simulink model "mdlspol2pop"  (Simulink 7.8)
settings: Solver=ode45  StartTime=0.0  StopTime=500  RelTol=1e-3
settings Model: Creator=polacmi1  LastModifiedBy=polacekm
settings GRTTargetCC: CombineOutputUpdateFcns=on

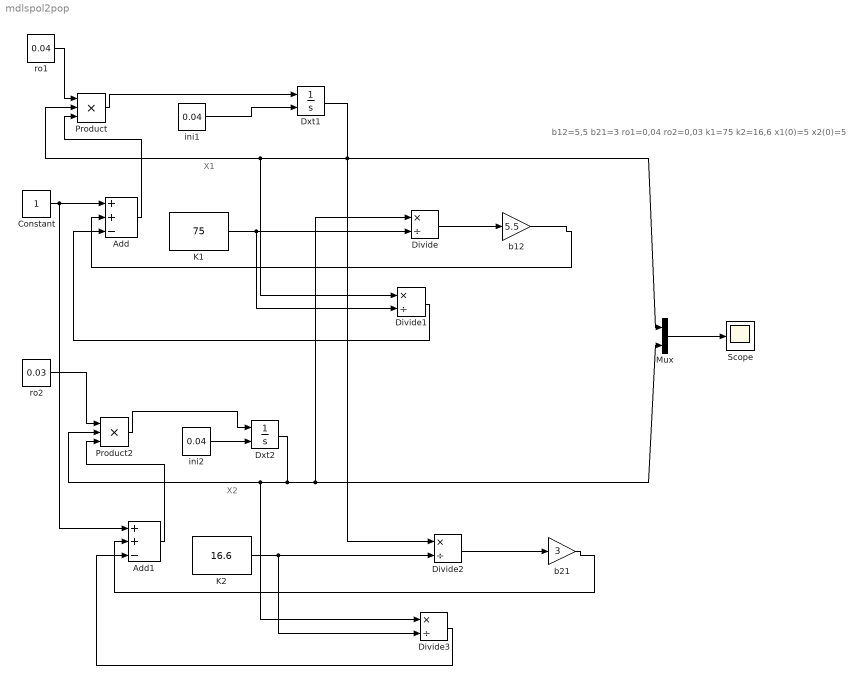
== system mdlspol2pop ==
  note: X1
  note: X2
  note: b12=5,5
      | b21=3
      | ro1=0,04
      | ro2=0,03
      | k1=75
      | k2=16,6
      | x1(0)=5
      | x2(0)=5
  Add : Sum  Inputs=++-
  Add1 : Sum  Inputs=++-
  Constant : Constant
  Divide{,1..3} (4 alike) : Product  Inputs=*/
  Dxt1 : Integrator  InitialConditionSource=external  InitialCondition=10
  Dxt2 : Integrator  InitialConditionSource=external  InitialCondition=10
  K1 : Constant  Value=75
  K2 : Constant  Value=16.6
  Mux : Mux  Inputs=2
  Product : Product  Inputs=3  RndMeth=Zero
  Product2 : Product  Inputs=3  RndMeth=Zero
  Scope : Scope
      settings: SaveName=sc
  b12 : Gain  Gain=5.5
  b21 : Gain  Gain=3
  ini1 : Constant  Value=0.04
  ini2 : Constant  Value=0.04
  ro1 : Constant  Value=0.04
  ro2 : Constant  Value=0.03
  wires:
  Dxt1/1 -> Product/2, Divide1/1, Divide2/1, Mux/1
  ro1/1 -> Product/1
  Product/1 -> Dxt1/1
  Constant/1 -> Add/1, Add1/1
  K1/1 -> Divide/2, Divide1/2
  Divide1/1 -> Add/3
  Add/1 -> Product/3
  b12/1 -> Add/2
  Dxt2/1 -> Product2/2, Divide3/1, Divide/1, Mux/2
  ro2/1 -> Product2/1
  Product2/1 -> Dxt2/1
  K2/1 -> Divide3/2, Divide2/2
  Divide3/1 -> Add1/3
  Add1/1 -> Product2/3
  Divide2/1 -> b21/1
  b21/1 -> Add1/2
  Divide/1 -> b12/1
  Mux/1 -> Scope/1
  ini1/1 -> Dxt1/2
  ini2/1 -> Dxt2/2
